simulink model "BicycleModel"  (Simulink 8.6)
settings: Solver=VariableStepAuto  StartTime=0.0  StopTime=inf  RelTol=1e-3
settings Model: Creator=Oscar  LastModifiedBy=Oscar
settings DataIOCC: SaveFormat=Dataset  SignalLoggingSaveFormat=Dataset
settings OptimizationCC: ExpressionDepthLimit=128
settings DebuggingCC: UnderspecifiedInitializationDetection=Simplified  MergeDetectMultiDrivingBlocksExec=error  SolverPrmCheckMsg=none  FcnCallInpInsideContextMsg=EnableAllAsError  StateNameClashWarn=none
settings HardwareCC: ProdBitPerPointer=64  ProdLargestAtomicFloat=Float  ProdIntDivRoundTo=Zero  ProdEndianess=LittleEndian  ProdWordSize=64  ProdHWDeviceType=Intel->x86-64 (Windows64)
settings GRTTargetCC: GeneratePreprocessorConditionals=Use local settings  CombineOutputUpdateFcns=on  GRTInterface=off
settings ConfigComp: CovModelRefEnable=off

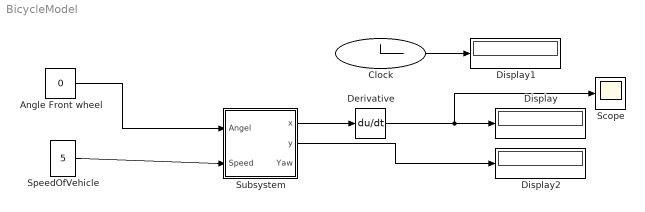
== system BicycleModel ==
  Angle Front wheel : Constant  Value=0
  Clock : Clock
      settings: Decimation=1000
  Derivative : Derivative
  Display : Display
  Display1 : Display
  Display2 : Display
  Scope : Scope
  SpeedOfVehicle : Constant  Value=5
  Subsystem : Subsystem
  wires:
  Angle Front wheel/1 -> Subsystem/1(Angel)
  SpeedOfVehicle/1 -> Subsystem/2(Speed)
  Clock/1 -> Display1/1
  Subsystem/1(x) -> Derivative/1
  Subsystem/2(y) -> Display2/1
  Derivative/1 -> Scope/1, Display/1

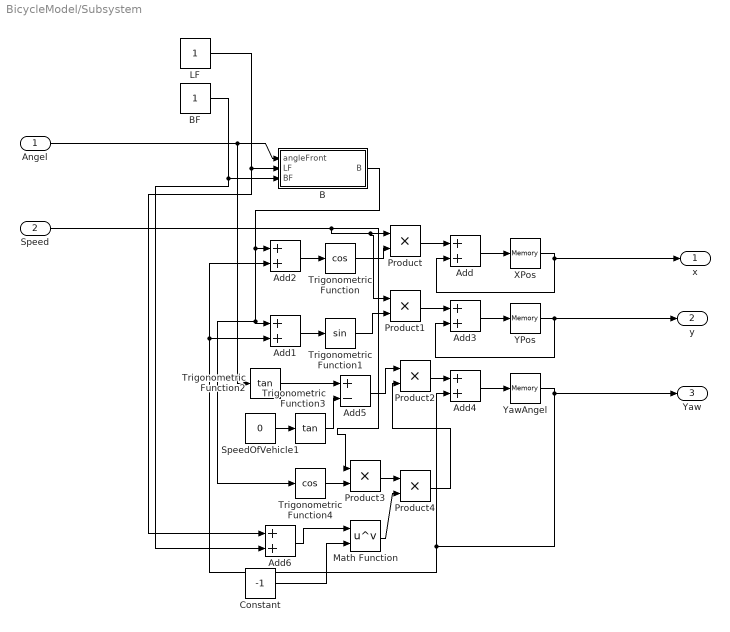
== system BicycleModel/Subsystem ==
  Angel : Inport
  Speed : Inport  Port=2
  Add{,1..4,6} (6 alike) : Sum
  Add5 : Sum  Inputs=+-
  B : Subsystem
  BF : Constant
  Constant : Constant  Value=-1
  LF : Constant
  Math Function : Math  Operator=pow  SaturateOnIntegerOverflow=on
  Product{,1..4} (5 alike) : Product
  SpeedOfVehicle1 : Constant  Value=0
  Trigonometric Function : Trigonometry  Operator=cos
  Trigonometric Function1 : Trigonometry
  Trigonometric Function2 : Trigonometry  Operator=tan
  Trigonometric Function3 : Trigonometry  Operator=tan
  Trigonometric Function4 : Trigonometry  Operator=cos
  XPos : Memory  InheritSampleTime=on  LinearizeMemory=on
  YPos : Memory  InheritSampleTime=on  LinearizeMemory=on
  YawAngel : Memory  X0=pi/2  InheritSampleTime=on  LinearizeMemory=on
  x : Outport
  y : Outport  Port=2
  Yaw : Outport  Port=3
  wires:
  Trigonometric Function2/1 -> Add5/1
  Add/1 -> XPos/1
  Add2/1 -> Trigonometric Function/1
  Product1/1 -> Add3/1
  Product4/1 -> Product2/2
  Add4/1 -> YawAngel/1
  Add1/1 -> Trigonometric Function1/1
  Trigonometric Function4/1 -> Product3/2
  YPos/1 -> y/1, Add3/2
  YawAngel/1 -> Yaw/1, Add4/2, Add2/2, Add1/2
  Trigonometric Function/1 -> Product/2
  Trigonometric Function3/1 -> Add5/2
  Product/1 -> Add/1
  Trigonometric Function1/1 -> Product1/2
  Product3/1 -> Product4/1
  SpeedOfVehicle1/1 -> Trigonometric Function3/1
  Add3/1 -> YPos/1
  Add5/1 -> Product2/1
  Angel/1 -> Trigonometric Function2/1, B/1(angleFront)
  XPos/1 -> x/1, Add/2
  Product2/1 -> Add4/1
  LF/1 -> Add6/1, B/2(LF)
  Math Function/1 -> Product4/2
  Speed/1 -> Product3/1, Product1/1, Product/1
  BF/1 -> Add6/2, B/3(BF)
  Add6/1 -> Math Function/1
  Constant/1 -> Math Function/2
  B/1(B) -> Trigonometric Function4/1, Add1/1, Add2/1

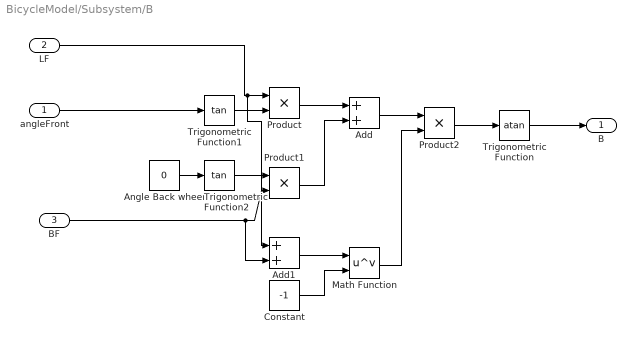
== system BicycleModel/Subsystem/B ==
  angleFront : Inport
  LF : Inport  Port=2
  BF : Inport  Port=3
  Add : Sum
  Add1 : Sum
  Angle Back wheel : Constant  Value=0
  Constant : Constant  Value=-1
  Math Function : Math  Operator=pow  SaturateOnIntegerOverflow=on
  Product : Product
  Product1 : Product
  Product2 : Product
  Trigonometric Function : Trigonometry  Operator=atan
  Trigonometric Function1 : Trigonometry  Operator=tan
  Trigonometric Function2 : Trigonometry  Operator=tan
  B : Outport
  wires:
  Angle Back wheel/1 -> Trigonometric Function2/1
  Trigonometric Function1/1 -> Product/2
  Add/1 -> Product2/1
  Trigonometric Function2/1 -> Product1/1
  Product1/1 -> Add/2
  Product/1 -> Add/1
  angleFront/1 -> Trigonometric Function1/1
  BF/1 -> Add1/2, Product1/2
  Math Function/1 -> Product2/2
  Add1/1 -> Math Function/1
  Constant/1 -> Math Function/2
  Trigonometric Function/1 -> B/1
  Product2/1 -> Trigonometric Function/1
  LF/1 -> Add1/1, Product/1
